simulink library "fixpt_lib_4"  (Simulink 6.0)
settings: Solver=ode45  SolverMode=SingleTasking  StartTime=0.0  StopTime=10.0  RelTol=1e-3
undefined symbols (not defined in the file or in its folder): DiscIntNeverNeededParam, NumBits1, NumBits2, Slope1, Slope2
libraries: simulink x112, simulink_need_slupdate x1
settings Model: CovMetricSettings=d  Creator=andyb  LastModifiedBy=dyang  ExtModeAutoUpdateStatusClock=off  ProdHWDeviceType=Specified
settings Model: ForwardingTableString=|
  | ||__slOldName__||fixpt_lib_4/LookUp/Cosine/Handle Quarter Symmetry Cosine||__slNewName__||simulink/Lookup
  | Tables/Cosine/Handle Quarter Symmetry Cosine||__slOldName__||fixpt_lib_4/LookUp/Sine/Handle Quarter Symmetry Sine||__slNewName__||simulink/Lookup
  | Tables/Sine/Handle Quarter Symetery Sine

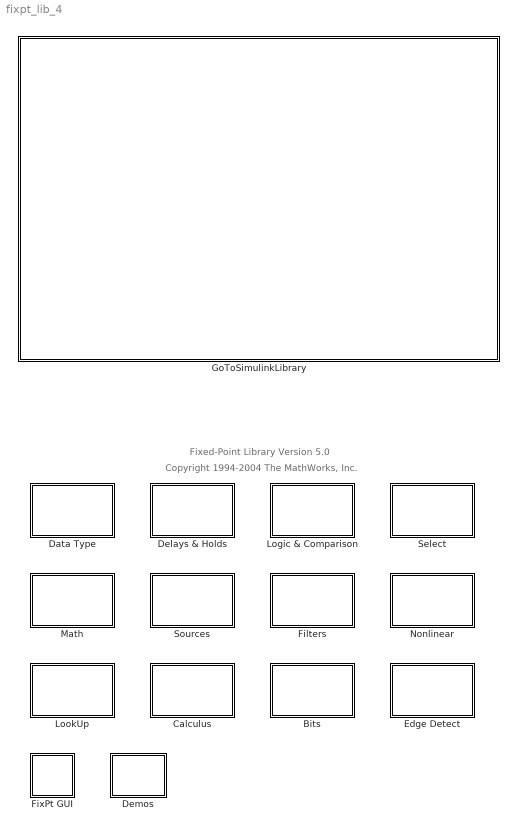
== system fixpt_lib_4 ==
  note: Fixed-Point Library Version 5.0
  note: Copyright 1994-2004 The MathWorks, Inc.
  Bits : Subsystem  PropExecContextAcrossSSBoundary=on
      mask Display: disp('Bits')
  Calculus : Subsystem  PropExecContextAcrossSSBoundary=on
      mask Display: disp('Calculus')
  Data Type : Subsystem  PropExecContextAcrossSSBoundary=on
      mask Display: disp('Data Type\nConversion &\nPropagation')
  Delays & Holds : Subsystem  PropExecContextAcrossSSBoundary=on
      mask Display: disp('Delays\n& Holds')
  Demos : Subsystem  PropExecContextAcrossSSBoundary=on
      settings: OpenFcn=demo('blocksets','Fixed Point')
      mask Help: fpbhelp
      mask Display: disp('Demos')
  Edge Detect : Subsystem  PropExecContextAcrossSSBoundary=on
      mask Display: disp('Edge\nDetect')
  Filters : Subsystem  PropExecContextAcrossSSBoundary=on
      mask Display: disp('Filters')
  FixPt GUI : Subsystem  PropExecContextAcrossSSBoundary=on
      settings: OpenFcn=fxptdlg(bdroot)
      mask Type: Fixed-Point GUI
      mask Description: Fixed point GUI block.
      mask Help: fpbhelp('fixptgui');
      mask Display: disp('FixPt\nGUI')
  GoToSimulinkLibrary : Subsystem  PropExecContextAcrossSSBoundary=on  mask(GoToSimulinkLibrary){}
      mask init:
      | dispstr = [...
      | 'This is an obsolete library. All blocks previously from\n',...
      | 'Fixed-Point Blockset are automatically mapped to\n',...
      | 'unified blocks in the main Simulink library.\n\n', ...
      | 'DOUBLE CLICK HERE to open the main Simulink library.\n\n',...
      | 'Unified blocks support both floating-point and fixed-point\ndata types.  ',...
      | 'When used with floating-point or built-in\n',...
      | 'integer types, an extra license is not required.\n\n', ...
      | 'Simulink Fixed Point has replaced Fixed-Point Blockset.\n',...
      | 'It provides fixed-point capabilities across the Simulink\n',...
      | 'toolchain including: Simulink Blocks, Stateflow,\n',...
      | 'Signal Processing Blockset, Real-Time Workshop,\n',...
      | 'and other code generation tools.'];
      settings: OpenFcn=fixpt;
      mask Display: disp(dispstr)
  Logic & Comparison : Subsystem  PropExecContextAcrossSSBoundary=on
      mask Display: disp('Logic &\nComparison')
  LookUp : Subsystem  PropExecContextAcrossSSBoundary=on
      mask Display: disp('Look-Up Tables')
  Math : Subsystem  PropExecContextAcrossSSBoundary=on
      mask Display: disp('Math')
  Nonlinear : Subsystem  PropExecContextAcrossSSBoundary=on
      mask Display: disp('Nonlinear')
  Select : Subsystem  PropExecContextAcrossSSBoundary=on
      mask Display: disp('Select')
  Sources : Subsystem  PropExecContextAcrossSSBoundary=on
      mask Display: disp('Sources')

== system fixpt_lib_4/Bits ==
  note: Copyright 1994-2004 The MathWorks, Inc.
  note: Fixed-Point Library Version 5.0
  Bit Clear : simulink/Logic and Bit Operations/Bit Clear  iBit=0
  Bit Set : simulink/Logic and Bit Operations/Bit Set  iBit=0
  Bitwise Operator : simulink/Logic and Bit Operations/Bitwise Operator  logicop=AND  UseBitMask=on  BitMask=bin2dec('11011001')  BitMaskRealWorld=Stored Integer
  Examples : Subsystem  PropExecContextAcrossSSBoundary=on
      mask Display: disp('Bitwise\nExamples')
  Shift Arithmetic : simulink/Logic and Bit Operations/Shift Arithmetic  nBitShiftRight=8  nBinPtShiftRight=0

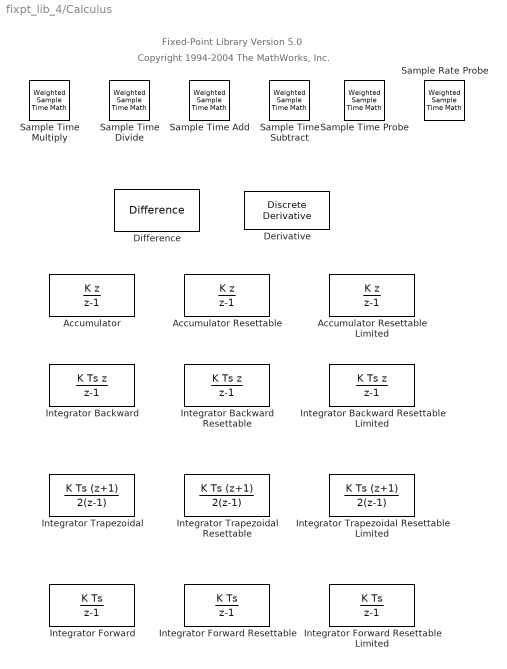
== system fixpt_lib_4/Calculus ==
  note: Fixed-Point Library Version 5.0
  note: Copyright 1994-2004 The MathWorks, Inc.
  Accumulator : DiscreteIntegrator  IntegratorMethod=Accumulation: Backward Euler  InitialConditionMode=State only (most efficient)  SampleTime=-1  ICPrevOutput=DiscIntNeverNeededParam  ICPrevScaledInput=DiscIntNeverNeededParam
  Accumulator Resettable : DiscreteIntegrator  IntegratorMethod=Accumulation: Backward Euler  ExternalReset=level  SampleTime=-1  ICPrevOutput=DiscIntNeverNeededParam  ICPrevScaledInput=DiscIntNeverNeededParam
  Accumulator Resettable Limited : DiscreteIntegrator  IntegratorMethod=Accumulation: Backward Euler  ExternalReset=level  SampleTime=-1  LimitOutput=on  UpperSaturationLimit=0.5  LowerSaturationLimit=-0.5  ICPrevOutput=DiscIntNeverNeededParam  ICPrevScaledInput=DiscIntNeverNeededParam
  Derivative : simulink/Discrete/Discrete Derivative  gainval=1.0  ICPrevScaledInput=0.0  OutDataType=sfix(16)  OutScaling=2^-10  DoSatur=off
  Difference : simulink/Discrete/Difference  ICPrevInput=0.0  OutDataType=sfix(16)  OutScaling=2^-10  DoSatur=off
  Integrator Backward : DiscreteIntegrator  IntegratorMethod=Integration: Backward Euler  InitialConditionMode=State only (most efficient)  SampleTime=-1  ICPrevOutput=DiscIntNeverNeededParam  ICPrevScaledInput=DiscIntNeverNeededParam
  Integrator Backward Resettable : DiscreteIntegrator  IntegratorMethod=Integration: Backward Euler  ExternalReset=level  SampleTime=-1  ICPrevOutput=DiscIntNeverNeededParam  ICPrevScaledInput=DiscIntNeverNeededParam
  Integrator Backward Resettable Limited : DiscreteIntegrator  IntegratorMethod=Integration: Backward Euler  ExternalReset=level  SampleTime=-1  LimitOutput=on  UpperSaturationLimit=0.5  LowerSaturationLimit=-0.5  ICPrevOutput=DiscIntNeverNeededParam  ICPrevScaledInput=DiscIntNeverNeededParam
  Integrator Forward : DiscreteIntegrator  InitialConditionMode=State only (most efficient)  SampleTime=-1  ICPrevOutput=DiscIntNeverNeededParam  ICPrevScaledInput=DiscIntNeverNeededParam
  Integrator Forward Resettable : DiscreteIntegrator  ExternalReset=level  InitialConditionMode=State only (most efficient)  SampleTime=-1  ICPrevOutput=DiscIntNeverNeededParam  ICPrevScaledInput=DiscIntNeverNeededParam
  Integrator Forward Resettable Limited : DiscreteIntegrator  ExternalReset=level  InitialConditionMode=State only (most efficient)  SampleTime=-1  LimitOutput=on  UpperSaturationLimit=0.5  LowerSaturationLimit=-0.5  ICPrevOutput=DiscIntNeverNeededParam  ICPrevScaledInput=DiscIntNeverNeededParam
  Integrator Trapezoidal : DiscreteIntegrator  IntegratorMethod=Integration: Trapezoidal  InitialConditionMode=State only (most efficient)  SampleTime=-1  ICPrevOutput=DiscIntNeverNeededParam  ICPrevScaledInput=DiscIntNeverNeededParam
  Integrator Trapezoidal Resettable : DiscreteIntegrator  IntegratorMethod=Integration: Trapezoidal  ExternalReset=level  SampleTime=-1  ICPrevOutput=DiscIntNeverNeededParam  ICPrevScaledInput=DiscIntNeverNeededParam
  Integrator Trapezoidal Resettable Limited : DiscreteIntegrator  IntegratorMethod=Integration: Trapezoidal  ExternalReset=level  SampleTime=-1  LimitOutput=on  UpperSaturationLimit=0.5  LowerSaturationLimit=-0.5  ICPrevOutput=DiscIntNeverNeededParam  ICPrevScaledInput=DiscIntNeverNeededParam
  Sample Rate Probe : simulink/Math Operations/Weighted Sample Time Math  TsampMathOp=1/Ts Only  weightValue=1  TsampMathImp=Online Calculations  DoSatur=off
  Sample Time Add : simulink/Math Operations/Weighted Sample Time Math  TsampMathOp=+  weightValue=1.0  TsampMathImp=Online Calculations  DoSatur=off
  Sample Time Divide : simulink/Math Operations/Weighted Sample Time Math  TsampMathOp=/  weightValue=1.0  TsampMathImp=Online Calculations  DoSatur=off
  Sample Time Multiply : simulink/Math Operations/Weighted Sample Time Math  TsampMathOp=*  weightValue=1.0  TsampMathImp=Online Calculations  DoSatur=off
  Sample Time Probe : simulink/Math Operations/Weighted Sample Time Math  TsampMathOp=Ts Only  weightValue=1.0  TsampMathImp=Online Calculations  DoSatur=off
  Sample Time Subtract : simulink/Math Operations/Weighted Sample Time Math  TsampMathOp=-  weightValue=1.0  TsampMathImp=Online Calculations  DoSatur=off

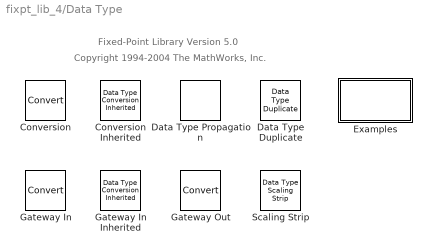
== system fixpt_lib_4/Data Type ==
  note: Fixed-Point Library Version 5.0
  note: Copyright 1994-2004 The MathWorks, Inc.
  Conversion : DataTypeConversion  OutDataTypeMode=Specify via dialog  OutScaling=2^-10
  Conversion Inherited : simulink/Signal Attributes/Data Type Conversion Inherited  ConvertRealWorld=Real World Value  DoSatur=off
  Data Type Duplicate : simulink/Signal Attributes/Data Type Duplicate  NumInputPorts=2
  Data Type Propagation : simulink/Signal Attributes/Data Type Propagation  PropDataType=sfix(16)  IfRefDouble=double  IfRefSingle=single  IsSigned=IsSigned1 or IsSigned2  NumBitsBase=max([NumBits1 NumBits2])  NumBitsMult=1  NumBitsAdd=0  NumBitsAllowFinal=1:128  PropScaling=2^-10  ValuesUsedBestPrec=[5 -7]  SlopeBase=min([Slope1 Slope2])  SlopeMult=1  SlopeAdd=0  BiasBase=Bias1  BiasMult=1  BiasAdd=0
  Examples : Subsystem  PropExecContextAcrossSSBoundary=on
      settings: OpenFcn=open_system('fixpt_dtprop')
      mask Display: disp('Data Type\nPropagation\nExamples')
  Gateway In : DataTypeConversion  OutDataTypeMode=Specify via dialog  OutScaling=2^-10
  Gateway In Inherited : simulink/Signal Attributes/Data Type Conversion Inherited  ConvertRealWorld=Real World Value  DoSatur=off
  Gateway Out : DataTypeConversion  OutDataTypeMode=double
  Scaling Strip : simulink/Signal Attributes/Data Type Scaling Strip

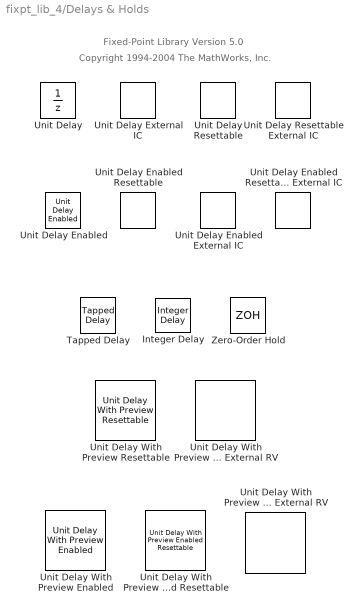
== system fixpt_lib_4/Delays & Holds ==
  note: Copyright 1994-2004 The MathWorks, Inc.
  note: Fixed-Point Library Version 5.0
  Integer Delay : simulink/Discrete/Integer Delay  vinit=0.0  samptime=-1  NumDelays=4
  Tapped Delay : simulink/Discrete/Tapped Delay  vinit=0.0  samptime=-1  NumDelays=4  DelayOrder=Oldest  includeCurrent=off
  Unit Delay : UnitDelay  X0=0.0  SampleTime=-1
  Unit Delay Enabled : simulink/Additional Math & Discrete/Additional Discrete/Unit Delay Enabled  vinit=0.0  tsamp=-1
  Unit Delay Enabled External IC : simulink/Additional Math & Discrete/Additional Discrete/Unit Delay Enabled External IC  tsamp=-1
  Unit Delay Enabled Resettable : simulink/Additional Math & Discrete/Additional Discrete/Unit Delay Enabled Resettable  vinit=0.0  tsamp=-1
  Unit Delay Enabled Resettable External IC : simulink/Additional Math & Discrete/Additional Discrete/Unit Delay Enabled Resettable External IC  tsamp=-1
  Unit Delay External IC : simulink/Additional Math & Discrete/Additional Discrete/Unit Delay External IC  tsamp=-1
  Unit Delay Resettable : simulink/Additional Math & Discrete/Additional Discrete/Unit Delay Resettable  vinit=0.0  tsamp=-1
  Unit Delay Resettable External IC : simulink/Additional Math & Discrete/Additional Discrete/Unit Delay Resettable External IC  tsamp=-1
  Unit Delay With Preview Enabled : simulink/Additional Math & Discrete/Additional Discrete/Unit Delay With Preview Enabled  vinit=0.0  tsamp=-1
  Unit Delay With Preview Enabled Resettable : simulink/Additional Math & Discrete/Additional Discrete/Unit Delay With Preview Enabled Resettable  vinit=0.0  tsamp=-1
  Unit Delay With Preview Enabled Resettable External RV : simulink/Additional Math & Discrete/Additional Discrete/Unit Delay With Preview Enabled Resettable External RV  vinit=0.0  tsamp=-1
  Unit Delay With Preview Resettable : simulink/Additional Math & Discrete/Additional Discrete/Unit Delay With Preview Resettable  vinit=0.0  tsamp=-1
  Unit Delay With Preview Resettable External RV : simulink/Additional Math & Discrete/Additional Discrete/Unit Delay With Preview Resettable External RV  vinit=0.0  tsamp=-1
  Zero-Order Hold : ZeroOrderHold

== system fixpt_lib_4/Demos ==

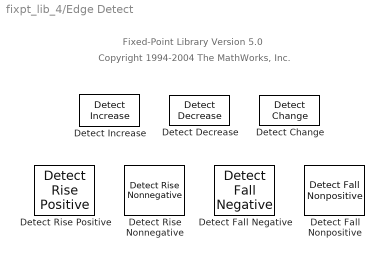
== system fixpt_lib_4/Edge Detect ==
  note: Fixed-Point Library Version 5.0
  note: Copyright 1994-2004 The MathWorks, Inc.
  Detect Change : simulink/Logic and Bit Operations/Detect Change  vinit=0
  Detect Decrease : simulink/Logic and Bit Operations/Detect Decrease  vinit=0.0
  Detect Increase : simulink/Logic and Bit Operations/Detect Increase  vinit=0.0
  Detect Fall Negative : simulink/Logic and Bit Operations/Detect Fall Negative  vinit=0
  Detect Fall Nonpositive : simulink/Logic and Bit Operations/Detect Fall Nonpositive  vinit=0
  Detect Rise Nonnegative : simulink/Logic and Bit Operations/Detect Rise Nonnegative  vinit=0
  Detect Rise Positive : simulink/Logic and Bit Operations/Detect Rise Positive  vinit=0

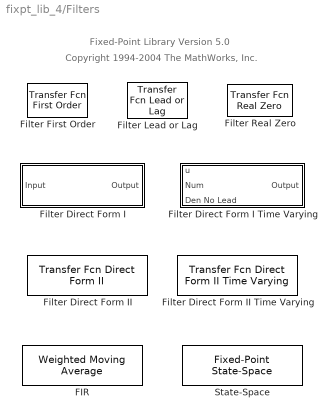
== system fixpt_lib_4/Filters ==
  note: Copyright 1994-2004 The MathWorks, Inc.
  note: Fixed-Point Library Version 5.0
  FIR : simulink/Discrete/Weighted Moving Average  mgainval=[0.1:0.1:1 0.9:-0.1:0.1]  vinit=0.0  samptime=-1  GainDataType=sfix( 16 )  MatRadixGroup=Best Precision: Matrix-wise  GainScaling=2^-10  OutDataType=sfix(16)  OutScaling=2^-10  DoSatur=off
  Filter Direct Form I : Subsystem  PropExecContextAcrossSSBoundary=on  mask(Transfer Fcn Direct Form I){NumCoefVec=[0.2 0.3 0.2], DenCoefVec=[-0.9    0.6], ICPrevOutput=0.0, ICPrevInput=0.0, RndMeth=Floor, DoSatur=off}
      mask prompts: NumCoefVec "Numerator coefficients:"; DenCoefVec "Denominator coefficients excluding lead (which must be 1.0):"; ICPrevOutput "Initial condition for previous output:"; ICPrevInput "Initial condition for previous input:"; RndMeth "Round toward:"; DoSatur "Saturate to max or min when overflows occur"
      mask help:
      | A Direct Form I realization of the specified transfer is used.  Only single input single output transfer functions are supported.
      |
      | The data types and scalings of the output, the coefficients, and any temporary variables are automatically selected.  The automatic choices will be acceptable in many situations.  In situations where the automatic choices give unacceptable results, manual layout of the filter is necessary.  For manual layout, it is suggested that the blocks under this mask be used as a starting point.
      |
      | Note 1:
      | The full denominator should have a leading coefficient of +1.0, but this leading coefficient should be excluded when entering the parameter.  For example, if the denominator is
      |   den =
      |             1         -1.7         0.72
      | just enter
      |   den(2:end)  =
      |          -1.7         0.72
      |
      | Note 2:
      | The numerator does NOT need to be the same size as the full denominator.
      mask init:
      | blkH = gcbh;
      | blkName = getfullname(blkH);
      | 
      | vRndMeth = get_param(blkH,'RndMeth');
      | vDoSatur = get_param(blkH,'DoSatur');
      | DCGain = polyval(NumCoefVec,1)./polyval([1 DenCoefVec],1);
      | maxGain = max( 1, max(max(abs(DCGain))) );
      | maxGain = max( maxGain, abs(NumCoefVec(1)) );
      | OutputSlopeMult = 2^ceil(log2(maxGain));
      | 
      | set_param([blkName,'/NumCoef'],'RndMeth',vRndMeth, ...
      | 	'DoSatur',vDoSatur);
      | set_param([blkName,'/DenCoef'],'RndMeth',vRndMeth, ...
      | 	'DoSatur',vDoSatur);
      | set_param([blkName,'/Downcast'],'RndMeth',vRndMeth, ...
      | 	'DoSatur',vDoSatur);
      | set_param([blkName,'/Sum'],'RndMeth',vRndMeth, ...
      | 	'DoSatur',vDoSatur);
      mask StyleString: edit,edit,edit,edit,popup(Zero|Nearest|Ceiling|Floor),checkbox
      mask CallbackString: fixptdialog(gcbh)|fixptdialog(gcbh)||||
      mask Display: dpoly(NumCoefVec,[1 DenCoefVec],'z-')
  Filter Direct Form I Time Varying : Subsystem  PropExecContextAcrossSSBoundary=on  mask(Transfer Fcn Direct Form I Time Varying){ICPrevOutput=0.0, ICPrevInput=0.0, RndMeth=Floor, DoSatur=off}
      mask prompts: ICPrevOutput "Initial condition for previous output:"; ICPrevInput "Initial condition for previous input:"; RndMeth "Round toward:"; DoSatur "Saturate to max or min when overflows occur"
      mask help:
      | A Direct Form I realization of the specified transfer function is used.  Only single input single output transfer functions are supported.
      |
      | The data types and scalings of the output, the coefficients, and any temporary variables are automatically selected.  The automatic choices will be acceptable in many situations.  In situations where the automatic choices give unacceptable results, manual layout of the filter is necessary.  For manual layout, it is suggested that the blocks under this mask be used as a starting point.
      |
      | Note 1:
      | The full denominator should have a leading coefficient of +1.0, but this leading coefficient should be excluded when entering the parameter.  For example, if the denominator is
      |   den =
      |             1         -1.7         0.72
      | just enter
      |   den(2:end)  =
      |          -1.7         0.72
      |
      | Note 2:
      | The numerator does NOT need to be the same size as the full denominator.
      mask init:
      | blkH = gcbh;
      | blkName = getfullname(blkH);
      | 
      | vRndMeth = get_param(blkH,'RndMeth');
      | vDoSatur = get_param(blkH,'DoSatur');
      | set_param([blkName,'/Dot1'],'RndMeth',vRndMeth, ...
      | 	'DoSatur',vDoSatur);
      | set_param([blkName,'/Dot2'],'RndMeth',vRndMeth, ...
      | 	'DoSatur',vDoSatur);
      | set_param([blkName,'/Downcast'],'RndMeth',vRndMeth, ...
      | 	'DoSatur',vDoSatur);
      | set_param([blkName,'/Sum'],'RndMeth',vRndMeth, ...
      | 	'DoSatur',vDoSatur);
      mask StyleString: edit,edit,popup(Zero|Nearest|Ceiling|Floor),checkbox
      mask Display: fprintf('Direct\nForm I')
  Filter Direct Form II : simulink/Additional Math & Discrete/Additional Discrete/Transfer Fcn Direct Form II  NumCoefVec=[0.2 0.3 0.2]  DenCoefVec="[-0.9    0.6]"  vinit=0.0  DoSatur=off
  Filter Direct Form II Time Varying : simulink/Additional Math & Discrete/Additional Discrete/Transfer Fcn Direct Form II Time Varying  vinit=0.0  DoSatur=off
  Filter First Order : simulink/Discrete/Transfer Fcn First Order  PoleZ=0.95  ICPrevOutput=0.0  DoSatur=off
  Filter Lead or Lag : simulink/Discrete/Transfer Fcn Lead or Lag  PoleZ=0.95  ZeroZ=0.75  ICPrevOutput=0.0  ICPrevInput=0.0  DoSatur=off
  Filter Real Zero : simulink/Discrete/Transfer Fcn Real Zero  ZeroZ=0.75  ICPrevInput=0.0  DoSatur=off
  State-Space : simulink/Additional Math & Discrete/Additional Discrete/Fixed-Point State-Space  A=[2.6020 -2.2793 0.6708; 1 0 0; 0 1 0]  B=[ 1; 0; 0]  C="[0.0184    0.0024    0.0055]"  D=[0.0033]  X0=0.0  InternalDataType=float('double')  StateEqScaling=2^0  OutputEqScaling=2^0  DoSatur=off

== system fixpt_lib_4/FixPt GUI ==
  EmptySubSystem : Subsystem  PropExecContextAcrossSSBoundary=on

== system fixpt_lib_4/GoToSimulinkLibrary ==

== system fixpt_lib_4/Logic & Comparison ==
  note: Copyright 1994-2004 The MathWorks, Inc.
  note: Fixed-Point Library Version 5.0
  Compare To Constant : simulink/Logic and Bit Operations/Compare To Constant  relop=<=  const=3.0  LogicOutDataTypeMode=uint8
  Compare To Zero : simulink/Logic and Bit Operations/Compare To Zero  relop=<=  LogicOutDataTypeMode=uint8
  Examples : Subsystem  PropExecContextAcrossSSBoundary=on
      mask Display: disp('Logic &\nComparison\nExamples')
  Interval Test : simulink/Logic and Bit Operations/Interval Test  IntervalClosedRight=on  uplimit=0.5  IntervalClosedLeft=on  lowlimit=-0.5  LogicOutDataTypeMode=uint8
  Interval Test Dynamic : simulink/Logic and Bit Operations/Interval Test Dynamic  IntervalClosedRight=on  IntervalClosedLeft=on  LogicOutDataTypeMode=uint8
  Logical Operator : Logic  AllPortsSameDT=off  OutDataTypeMode=Specify via dialog
  Relational Operator : RelationalOperator  Operator=<=  LogicOutDataTypeMode=Specify via dialog  ZeroCross=off

== system fixpt_lib_4/LookUp ==
  note: Fixed-Point Library Version 5.0
  note: Copyright 1994-2004 The MathWorks, Inc.
  Cosine : simulink/Lookup Tables/Cosine  NumDataPoints=(2^5)+1
  Look-Up Table : Lookup  DialogController=Simulink.DDGSource  InputValues=-5:5  OutputValues=tanh([-5:5])  LookUpMeth=Interpolation-Use End Values  OutDataTypeMode=Specify via dialog  OutScaling=2^-10
  Look-Up Table Dynamic : simulink/Lookup Tables/Lookup Table Dynamic  LookUpMeth=Interpolation-Use End Values  OutputDataTypeScalingMode=Specify via dialog  OutDataType=sfix(16)  OutScaling=2^-10  DoSatur=off
  Look-Up Table (2-D) : Lookup2D  DialogController=Simulink.DDGSource  RowIndex=[1:3]  ColumnIndex=[1:3]  OutputValues=[4 5 6;16 19 20;10 18 23]  LookUpMeth=Interpolation-Use End Values  OutDataTypeMode=Specify via dialog  OutScaling=2^-10
  Sine : simulink/Lookup Tables/Sine  NumDataPoints=(2^5)+1

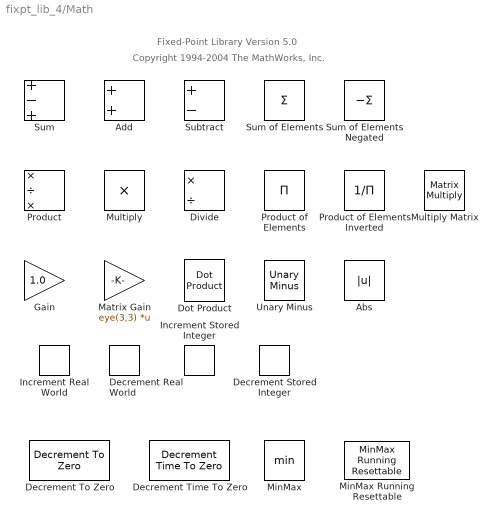
== system fixpt_lib_4/Math ==
  note: Copyright 1994-2004 The MathWorks, Inc.
  note: Fixed-Point Library Version 5.0
  Abs : Abs  ZeroCross=off
  Add : Sum  OutDataTypeMode=Specify via dialog  OutScaling=2^-10
  Decrement Real World : simulink/Additional Math & Discrete/Additional Math: Increment - Decrement/Decrement Real World
  Decrement Stored Integer : simulink/Additional Math & Discrete/Additional Math: Increment - Decrement/Decrement Stored Integer
  Decrement To Zero : simulink/Additional Math & Discrete/Additional Math: Increment - Decrement/Decrement To Zero
  Decrement Time To Zero : simulink/Additional Math & Discrete/Additional Math: Increment - Decrement/Decrement Time To Zero
  Divide : Product  Inputs=*/  OutDataTypeMode=Specify via dialog  OutScaling=2^-10
  Dot Product : simulink_need_slupdate/Dot Product  OutputDataTypeScalingMode=Specify via dialog  OutDataType=sfix(16)  OutScaling=2^-10  DoSatur=off
  Gain : Gain  Gain=1.0  ParameterDataTypeMode=Specify via dialog  ParameterScaling=2^-15  OutDataTypeMode=Specify via dialog  OutScaling=2^-10
  Increment Real World : simulink/Additional Math & Discrete/Additional Math: Increment - Decrement/Increment Real World
  Increment Stored Integer : simulink/Additional Math & Discrete/Additional Math: Increment - Decrement/Increment Stored Integer
  Matrix Gain : Gain  Gain=eye(3,3)  Multiplication=Matrix(K*u) (u vector)  ParameterDataTypeMode=Specify via dialog  ParameterDataType=sfix( 16 )  ParameterScaling=2^-10  OutDataTypeMode=Specify via dialog  OutScaling=2^-10
  MinMax : MinMax  OutScaling=2^-10  ZeroCross=off
  MinMax Running Resettable : simulink/Math Operations/MinMax Running Resettable  Function=min  vinit=0.0
  Multiply : Product  Inputs=**  OutDataTypeMode=Specify via dialog  OutScaling=2^-10
  Multiply Matrix : Product  Multiplication=Matrix(*)  OutDataTypeMode=Specify via dialog  OutScaling=2^-10
  Product : Product  Inputs=*/*  OutDataTypeMode=Specify via dialog  OutScaling=2^-10
  Product of Elements : Product  Inputs=*  OutDataTypeMode=Specify via dialog  OutScaling=2^-10
  Product of Elements Inverted : Product  Inputs=/  OutDataTypeMode=Specify via dialog  OutScaling=2^-10
  Subtract : Sum  Inputs=+-  OutDataTypeMode=Specify via dialog  OutScaling=2^-10
  Sum : Sum  Inputs=+-+  OutDataTypeMode=Specify via dialog  OutScaling=2^-10
  Sum of Elements : Sum  Inputs=+  OutDataTypeMode=Specify via dialog  OutScaling=2^-10
  Sum of Elements Negated : Sum  Inputs=-  OutDataTypeMode=Specify via dialog  OutScaling=2^-10
  Unary Minus : simulink/Math Operations/Unary Minus  DoSatur=off

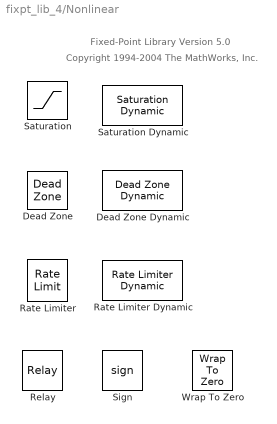
== system fixpt_lib_4/Nonlinear ==
  note: Copyright 1994-2004 The MathWorks, Inc.
  note: Fixed-Point Library Version 5.0
  Dead Zone : DeadZone  LowerValue=-1  UpperValue=1  LinearizeAsGain=off  ZeroCross=off
  Dead Zone Dynamic : simulink/Discontinuities/Dead Zone Dynamic
  Rate Limiter : RateLimiter  RisingSlewLimit=2  FallingSlewLimit=-2  SampleTimeMode=inherited
  Rate Limiter Dynamic : simulink/Discontinuities/Rate Limiter Dynamic
  Relay : Relay  OnSwitchValue=0  OffSwitchValue=0  OutputDataTypeScalingMode=Specify via dialog  OutDataType=uint(8)  OutScaling=2^-10  ConRadixGroup=Best Precision: Vector-wise
  Saturation : Saturate
  Saturation Dynamic : simulink/Discontinuities/Saturation Dynamic
  Sign : Signum  ZeroCross=off
  Wrap To Zero : simulink/Discontinuities/Wrap To Zero  Threshold=255

== system fixpt_lib_4/Select ==
  note: Copyright 1994-2004 The MathWorks, Inc.
  note: Fixed-Point Library Version 5.0
  Index Vector : MultiPortSwitch  Inputs=1  zeroidx=on
  MultiPort Switch : MultiPortSwitch  Inputs=3
  Switch : Switch  Threshold=1  ZeroCross=off

== system fixpt_lib_4/Sources ==
  note: Fixed-Point Library Version 5.0
  note: Copyright 1994-2004 The MathWorks, Inc.
  Constant : Constant  Value=0.0  OutDataTypeMode=Specify via dialog  ConRadixGroup=Best Precision: Vector-wise  OutScaling=2^-10
  Counter Free : simulink/Sources/Counter Free-Running  NumBits=16  tsamp=-1
  Counter Limited : simulink/Sources/Counter Limited  uplimit=7  tsamp=-1
  Repeating Sequence Interpolated : simulink/Sources/Repeating Sequence Interpolated  OutValues=[3 1 4 2 1].'  TimeValues=[0 0.1 0.5 0.6 1].'  LookUpMeth=Interpolation-Use End Values  tsamp=0.01  OutputDataTypeScalingMode=Specify via dialog  OutDataType=sfix(16)  OutScaling=2^-10
  Repeating Sequence Stair : simulink/Sources/Repeating Sequence Stair  OutValues=[3 1 4 2 1].'  tsamp=-1  OutputDataTypeScalingMode=Specify via dialog  OutDataType=sfix(16)  ConRadixGroup=Best Precision: Vector-wise  OutScaling=2^-12

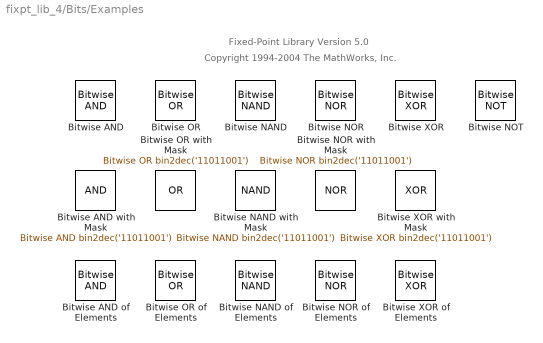
== system fixpt_lib_4/Bits/Examples ==
  note: Copyright 1994-2004 The MathWorks, Inc.
  note: Fixed-Point Library Version 5.0
  Bitwise AND : simulink/Logic and Bit Operations/Bitwise Operator  logicop=AND  UseBitMask=off  NumInputPorts=2  BitMask=bin2dec('11011001')  BitMaskRealWorld=Stored Integer
  Bitwise AND of Elements : simulink/Logic and Bit Operations/Bitwise Operator  logicop=AND  UseBitMask=off  BitMask=bin2dec('11011001')  BitMaskRealWorld=Stored Integer
  Bitwise AND with Mask : simulink/Logic and Bit Operations/Bitwise Operator  logicop=AND  UseBitMask=on  BitMask=bin2dec('11011001')  BitMaskRealWorld=Stored Integer
  Bitwise NAND : simulink/Logic and Bit Operations/Bitwise Operator  logicop=NAND  UseBitMask=off  NumInputPorts=2  BitMask=bin2dec('11011001')  BitMaskRealWorld=Stored Integer
  Bitwise NAND of Elements : simulink/Logic and Bit Operations/Bitwise Operator  logicop=NAND  UseBitMask=off  BitMask=bin2dec('11011001')  BitMaskRealWorld=Stored Integer
  Bitwise NAND with Mask : simulink/Logic and Bit Operations/Bitwise Operator  logicop=NAND  UseBitMask=on  BitMask=bin2dec('11011001')  BitMaskRealWorld=Stored Integer
  Bitwise NOR : simulink/Logic and Bit Operations/Bitwise Operator  logicop=NOR  UseBitMask=off  NumInputPorts=2  BitMask=bin2dec('11011001')  BitMaskRealWorld=Stored Integer
  Bitwise NOR of Elements : simulink/Logic and Bit Operations/Bitwise Operator  logicop=NOR  UseBitMask=off  BitMask=bin2dec('11011001')  BitMaskRealWorld=Stored Integer
  Bitwise NOR with Mask : simulink/Logic and Bit Operations/Bitwise Operator  logicop=NOR  UseBitMask=on  BitMask=bin2dec('11011001')  BitMaskRealWorld=Stored Integer
  Bitwise NOT : simulink/Logic and Bit Operations/Bitwise Operator  logicop=NOT  UseBitMask=off  BitMask=bin2dec('11011001')  BitMaskRealWorld=Stored Integer
  Bitwise OR : simulink/Logic and Bit Operations/Bitwise Operator  logicop=OR  UseBitMask=off  NumInputPorts=2  BitMask=bin2dec('11011001')  BitMaskRealWorld=Stored Integer
  Bitwise OR of Elements : simulink/Logic and Bit Operations/Bitwise Operator  logicop=OR  UseBitMask=off  BitMask=bin2dec('11011001')  BitMaskRealWorld=Stored Integer
  Bitwise OR with Mask : simulink/Logic and Bit Operations/Bitwise Operator  logicop=OR  UseBitMask=on  BitMask=bin2dec('11011001')  BitMaskRealWorld=Stored Integer
  Bitwise XOR : simulink/Logic and Bit Operations/Bitwise Operator  logicop=XOR  UseBitMask=off  NumInputPorts=2  BitMask=bin2dec('11011001')  BitMaskRealWorld=Stored Integer
  Bitwise XOR of Elements : simulink/Logic and Bit Operations/Bitwise Operator  logicop=XOR  UseBitMask=off  BitMask=bin2dec('11011001')  BitMaskRealWorld=Stored Integer
  Bitwise XOR with Mask : simulink/Logic and Bit Operations/Bitwise Operator  logicop=XOR  UseBitMask=on  BitMask=bin2dec('11011001')  BitMaskRealWorld=Stored Integer

== system fixpt_lib_4/Data Type/Examples ==

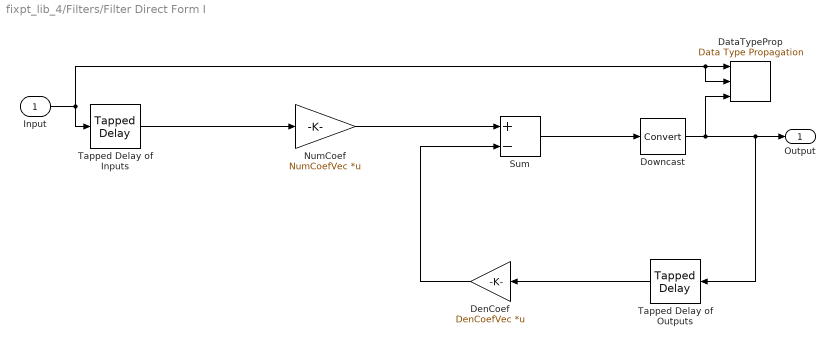
== system fixpt_lib_4/Filters/Filter Direct Form I ==
  Input : Inport  LatchInput=off
  DataTypeProp : simulink/Signal Attributes/Data Type Propagation  PropDataType=sfix(16)  IfRefDouble=double  IfRefSingle=single  IsSigned=IsSigned1 or IsSigned2  NumBitsBase=max([NumBits1 NumBits2])  NumBitsMult=1  NumBitsAdd=0  NumBitsAllowFinal=1:128  PropScaling=2^-10  ValuesUsedBestPrec=[5 -7]  SlopeBase=min([Slope1 Slope2])  SlopeMult=OutputSlopeMult  SlopeAdd=0  BiasBase=Bias1  BiasMult=0  BiasAdd=0
  DenCoef : Gain  Orientation=left  Gain=DenCoefVec  Multiplication=Matrix(K*u) (u vector)  ParameterDataType=float('double')  ParameterScalingMode=Use specified scaling  ParameterScaling=1  OutScaling=2^-10
      settings: AttributesFormatString=|
      | Data Type and Scaling Inherited
      | with goal of NO Quantization Noise
      | Possible Overflow or Saturation
  Downcast : DataTypeConversion  Description=|  OutDataType=float('double')  OutScaling=1  LockScale=on
      | Reduce from CPU Size
      |  to Global RAM Size
      settings: AttributesFormatString=%<Description>
  NumCoef : Gain  Gain=NumCoefVec  Multiplication=Matrix(K*u) (u vector)  ParameterDataType=float('double')  ParameterScalingMode=Use specified scaling  ParameterScaling=1  OutScaling=2^-10
      settings: AttributesFormatString=|
      | Data Type and Scaling Inherited
      | with goal of NO Quantization Noise
      | Possible Overflow or Saturation
  Sum : Sum  Tag=S16 2^-10  Inputs=+-  OutDataType=sfix(32)  OutScaling=2^(-26)  LockScale=on
      settings: AttributesFormatString=|
      | Data Type and Scaling Inherited
      | with goal of NO Quantization Noise
      | Possible Overflow or Saturation
  Tapped Delay of Inputs : simulink/Discrete/Tapped Delay  vinit=ICPrevInput  samptime=-1  NumDelays=-1  DelayOrder=Newest  includeCurrent=on
      settings: AttributesFormatString=|
      | Number of Taps
      | Inherited via Back Propagation
  Tapped Delay of Outputs : simulink/Discrete/Tapped Delay  Orientation=left  vinit=ICPrevOutput  samptime=-1  NumDelays=-1  DelayOrder=Newest  includeCurrent=off
      settings: AttributesFormatString=|
      | Number of Taps
      | Inherited via Back Propagation
  Output : Outport
  wires:
  Downcast/1 -> DataTypeProp/3, Tapped Delay of Outputs/1, Output/1
  Tapped Delay of Outputs/1 -> DenCoef/1
  DenCoef/1 -> Sum/2
  Sum/1 -> Downcast/1
  NumCoef/1 -> Sum/1
  Input/1 -> Tapped Delay of Inputs/1, DataTypeProp/2, DataTypeProp/1
  Tapped Delay of Inputs/1 -> NumCoef/1

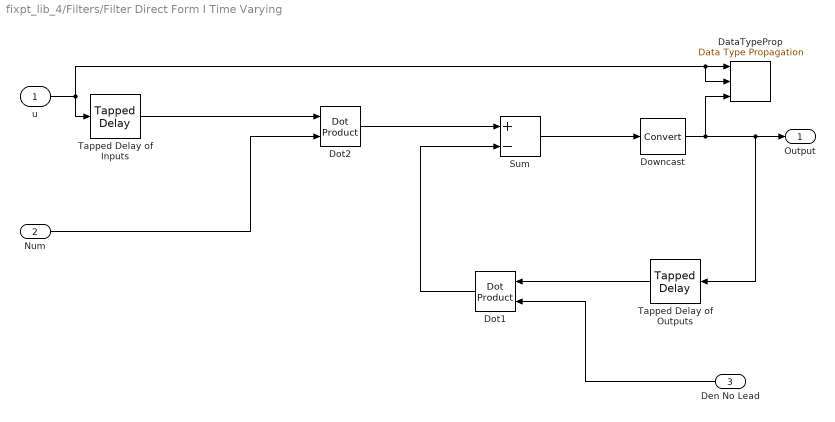
== system fixpt_lib_4/Filters/Filter Direct Form I Time Varying ==
  u : Inport  LatchInput=off
  Num : Inport  Port=2  LatchInput=off
  Den No Lead : Inport  Orientation=left  Port=3  LatchInput=off
  DataTypeProp : simulink/Signal Attributes/Data Type Propagation  PropDataType=sfix(16)  IfRefDouble=double  IfRefSingle=single  IsSigned=IsSigned1  NumBitsBase=NumBits1  NumBitsMult=1  NumBitsAdd=0  NumBitsAllowFinal=1:128  PropScaling=2^-10  ValuesUsedBestPrec=[5 -7]  SlopeBase=Slope1  SlopeMult=1  SlopeAdd=0  BiasBase=Bias1  BiasMult=1  BiasAdd=0
  Dot1 : simulink/Math Operations/Dot Product  Orientation=left  OutDataType=sfix(16)  OutScaling=2^-10  DoSatur=off
      settings: AttributesFormatString=|
      | Data Type and Scaling Inherited
      | with goal of NO Quantization Noise
      | Possible Overflow or Saturation
  Dot2 : simulink/Math Operations/Dot Product  OutDataType=sfix(16)  OutScaling=2^-10  DoSatur=off
      settings: AttributesFormatString=|
      | Data Type and Scaling Inherited
      | with goal of NO Quantization Noise
      | Possible Overflow or Saturation
  Downcast : DataTypeConversion  Description=|  OutDataType=float('double')  OutScaling=1  LockScale=on
      | Reduce from CPU Size
      |  to Global RAM Size
      settings: AttributesFormatString=%<Description>
  Sum : Sum  Tag=S16 2^-10  Inputs=+-  OutDataType=sfix(32)  OutScaling=2^(-26)  LockScale=on
      settings: AttributesFormatString=|
      | Data Type and Scaling Inherited
      | with goal of NO Quantization Noise
      | Possible Overflow or Saturation
  Tapped Delay of Inputs : simulink/Discrete/Tapped Delay  vinit=ICPrevInput  samptime=-1  NumDelays=-1  DelayOrder=Newest  includeCurrent=on
      settings: AttributesFormatString=|
      | Number of Taps
      | Inherited via Back Propagation
  Tapped Delay of Outputs : simulink/Discrete/Tapped Delay  Orientation=left  vinit=ICPrevOutput  samptime=-1  NumDelays=-1  DelayOrder=Newest  includeCurrent=off
      settings: AttributesFormatString=|
      | Number of Taps
      | Inherited via Back Propagation
  Output : Outport
  wires:
  Den No Lead/1 -> Dot1/2
  Num/1 -> Dot2/2
  Tapped Delay of Inputs/1 -> Dot2/1
  u/1 -> Tapped Delay of Inputs/1, DataTypeProp/2, DataTypeProp/1
  Dot2/1 -> Sum/1
  Sum/1 -> Downcast/1
  Dot1/1 -> Sum/2
  Tapped Delay of Outputs/1 -> Dot1/1
  Downcast/1 -> DataTypeProp/3, Output/1, Tapped Delay of Outputs/1

== system fixpt_lib_4/FixPt GUI/EmptySubSystem ==

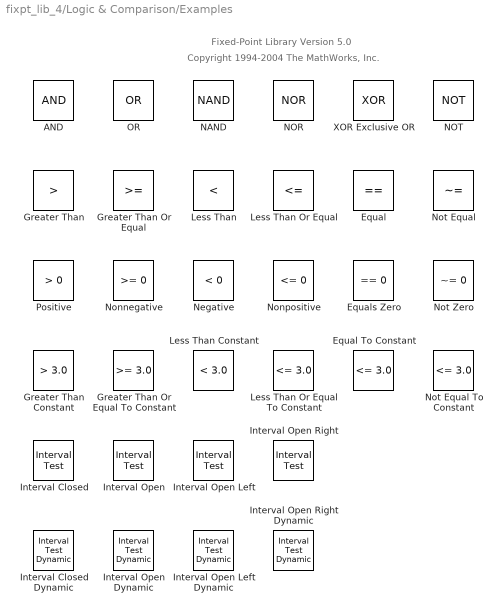
== system fixpt_lib_4/Logic & Comparison/Examples ==
  note: Fixed-Point Library Version 5.0
  note: Copyright 1994-2004 The MathWorks, Inc.
  AND : Logic  AllPortsSameDT=off  OutDataTypeMode=Specify via dialog
  Equal : RelationalOperator  Operator===  LogicOutDataTypeMode=Specify via dialog  ZeroCross=off
  Equal To Constant : simulink/Logic and Bit Operations/Compare To Constant  relop=<=  const=3.0  LogicOutDataTypeMode=uint8
  Equals Zero : simulink/Logic and Bit Operations/Compare To Zero  relop===  LogicOutDataTypeMode=uint8
  Greater Than : RelationalOperator  Operator=>  LogicOutDataTypeMode=Specify via dialog  ZeroCross=off
  Greater Than Constant : simulink/Logic and Bit Operations/Compare To Constant  relop=>  const=3.0  LogicOutDataTypeMode=uint8
  Greater Than Or Equal : RelationalOperator  LogicOutDataTypeMode=Specify via dialog  ZeroCross=off
  Greater Than Or Equal To Constant : simulink/Logic and Bit Operations/Compare To Constant  relop=>=  const=3.0  LogicOutDataTypeMode=uint8
  Interval Closed : simulink/Logic and Bit Operations/Interval Test  IntervalClosedRight=on  uplimit=0.5  IntervalClosedLeft=on  lowlimit=-0.5  LogicOutDataTypeMode=boolean
  Interval Closed Dynamic : simulink/Logic and Bit Operations/Interval Test Dynamic  IntervalClosedRight=on  IntervalClosedLeft=on  LogicOutDataTypeMode=boolean
  Interval Open : simulink/Logic and Bit Operations/Interval Test  IntervalClosedRight=off  uplimit=0.5  IntervalClosedLeft=off  lowlimit=-0.5  LogicOutDataTypeMode=boolean
  Interval Open Dynamic : simulink/Logic and Bit Operations/Interval Test Dynamic  IntervalClosedRight=off  IntervalClosedLeft=off  LogicOutDataTypeMode=boolean
  Interval Open Left : simulink/Logic and Bit Operations/Interval Test  IntervalClosedRight=on  uplimit=0.5  IntervalClosedLeft=off  lowlimit=-0.5  LogicOutDataTypeMode=boolean
  Interval Open Left Dynamic : simulink/Logic and Bit Operations/Interval Test Dynamic  IntervalClosedRight=on  IntervalClosedLeft=off  LogicOutDataTypeMode=boolean
  Interval Open Right : simulink/Logic and Bit Operations/Interval Test  IntervalClosedRight=off  uplimit=0.5  IntervalClosedLeft=on  lowlimit=-0.5  LogicOutDataTypeMode=boolean
  Interval Open Right Dynamic : simulink/Logic and Bit Operations/Interval Test Dynamic  IntervalClosedRight=off  IntervalClosedLeft=on  LogicOutDataTypeMode=boolean
  Less Than : RelationalOperator  Operator=<  LogicOutDataTypeMode=Specify via dialog  ZeroCross=off
  Less Than Constant : simulink/Logic and Bit Operations/Compare To Constant  relop=<  const=3.0  LogicOutDataTypeMode=uint8
  Less Than Or Equal : RelationalOperator  Operator=<=  LogicOutDataTypeMode=Specify via dialog  ZeroCross=off
  Less Than Or Equal To Constant : simulink/Logic and Bit Operations/Compare To Constant  relop=<=  const=3.0  LogicOutDataTypeMode=uint8
  NAND : Logic  Operator=NAND  AllPortsSameDT=off  OutDataTypeMode=Specify via dialog
  NOR : Logic  Operator=NOR  AllPortsSameDT=off  OutDataTypeMode=Specify via dialog
  NOT : Logic  Operator=NOT  Inputs=1  AllPortsSameDT=off  OutDataTypeMode=Specify via dialog
  Negative : simulink/Logic and Bit Operations/Compare To Zero  relop=<  LogicOutDataTypeMode=uint8
  Nonnegative : simulink/Logic and Bit Operations/Compare To Zero  relop=>=  LogicOutDataTypeMode=uint8
  Nonpositive : simulink/Logic and Bit Operations/Compare To Zero  relop=<=  LogicOutDataTypeMode=uint8
  Not Equal : RelationalOperator  Operator=~=  LogicOutDataTypeMode=Specify via dialog  ZeroCross=off
  Not Equal To Constant : simulink/Logic and Bit Operations/Compare To Constant  relop=<=  const=3.0  LogicOutDataTypeMode=uint8
  Not Zero : simulink/Logic and Bit Operations/Compare To Zero  relop=~=  LogicOutDataTypeMode=uint8
  OR : Logic  Operator=OR  AllPortsSameDT=off  OutDataTypeMode=Specify via dialog
  Positive : simulink/Logic and Bit Operations/Compare To Zero  relop=>  LogicOutDataTypeMode=uint8
  XOR Exclusive OR : Logic  Operator=XOR  AllPortsSameDT=off  OutDataTypeMode=Specify via dialog
